simulink model "Cascade_FIR"  (R2020b)
settings: Solver=VariableStepAuto  StartTime=0.0  StopTime=10.0  RelTol=1e-3
settings Model: Creator=DELL  LastModifiedBy=DELL
settings DataIOCC: SaveOutput=off  SaveTime=off

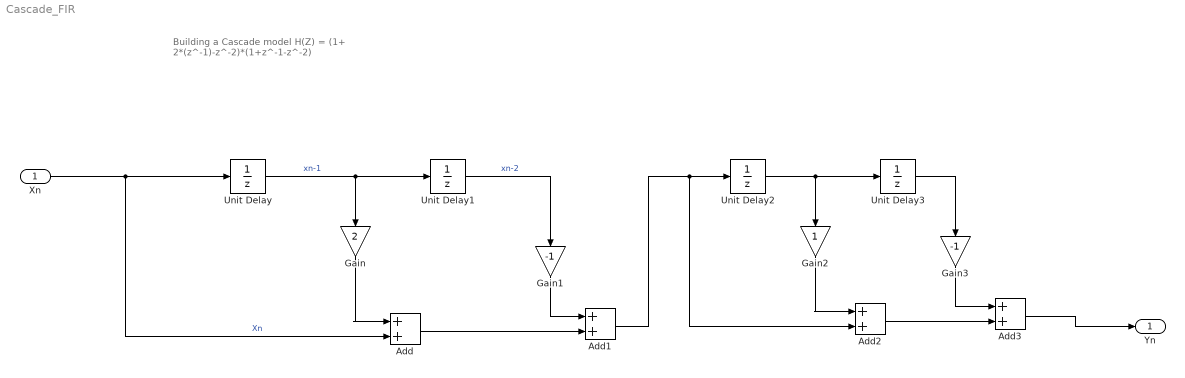
== system Cascade_FIR ==
  note: Building a Cascade model
      | H(Z) = (1+ 2*(z^-1)-z^-2)*(1+z^-1-z^-2)
  Xn : Inport  OutDataTypeStr=double  PortDimensions=1  SampleTime=[0,1]
  Add{,1..3} (4 alike) : Sum
  Gain : Gain  Gain=2
  Gain1 : Gain  Gain=-1
  Gain2 : Gain
  Gain3 : Gain  Gain=-1
  Unit Delay{,1..3} (4 alike) : UnitDelay  SampleTime=-1  HasFrameUpgradeWarning=on
  Yn : Outport  OutDataTypeStr=double  PortDimensions=1  SampleTime=[0,1]
  wires:
  Add1/1 -> Unit Delay2/1, Add2/2
  Unit Delay2/1 -> Unit Delay3/1, Gain2/1
  Unit Delay/1 -> Unit Delay1/1, Gain/1  "xn-1"
  Gain2/1 -> Add2/1
  Gain1/1 -> Add1/1
  Gain/1 -> Add/1
  Unit Delay3/1 -> Gain3/1
  Add3/1 -> Yn/1
  Unit Delay1/1 -> Gain1/1  "xn-2"
  Add/1 -> Add1/2
  Add2/1 -> Add3/2
  Gain3/1 -> Add3/1
  Xn/1 -> Unit Delay/1, Add/2  "Xn"
